simulink model "FCIACG_SIM"  (R2022a)
settings: Solver=VariableStepAuto  StartTime=0.0  StopTime=10.0  RelTol=1e-3
settings Model: Creator=Column  LastModifiedBy=Column

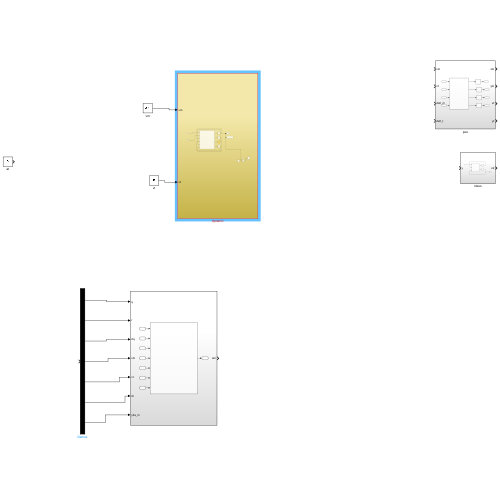
[thumbnail: Simulink's stored preview of the top-level diagram]
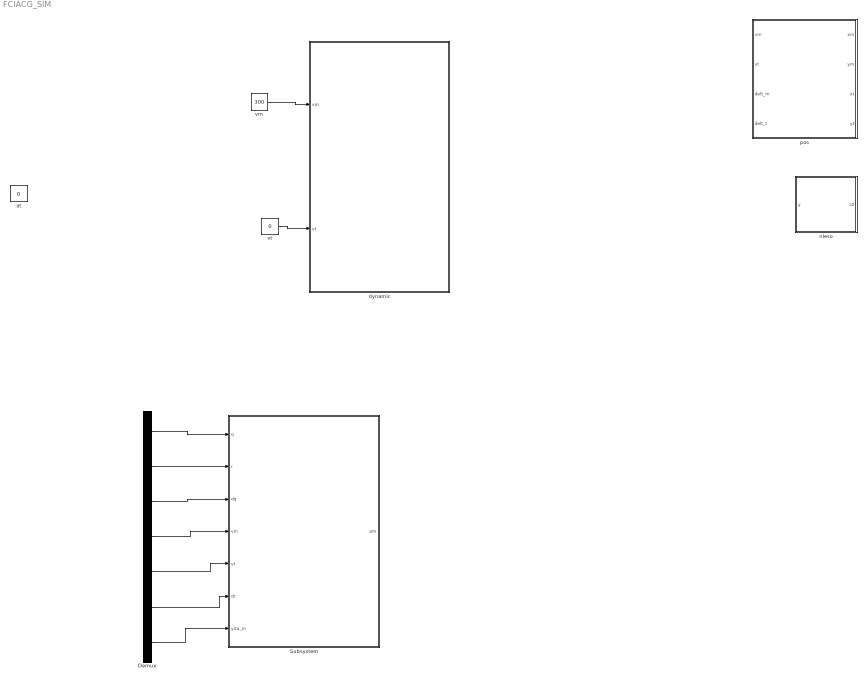
== system FCIACG_SIM ==
  Demux : Demux  Outputs=7
  Subsystem : Subsystem
  at : Constant  Value=0
  dynamic : Subsystem
  nleso : Subsystem
  pos : Subsystem
  vm : Constant  Value=300
  vt : Constant  Value=0
  wires:
  vm/1 -> dynamic/1(vm)
  Demux/1 -> Subsystem/1(q)
  Demux/2 -> Subsystem/2(r)
  Demux/3 -> Subsystem/3(dq)
  Demux/4 -> Subsystem/4(vm)
  Demux/5 -> Subsystem/5(vt)
  Demux/6 -> Subsystem/6(dr)
  Demux/7 -> Subsystem/7(yita_m)
  vt/1 -> dynamic/2(vt)

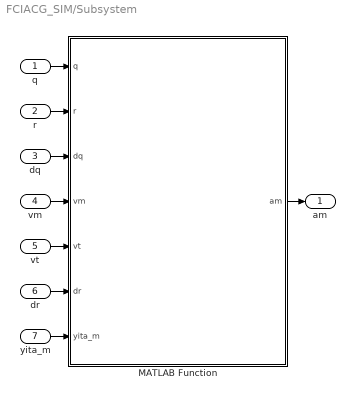
== system FCIACG_SIM/Subsystem ==
  q : Inport
  r : Inport  Port=2
  dq : Inport  Port=3
  vm : Inport  Port=4
  vt : Inport  Port=5
  dr : Inport  Port=6
  yita_m : Inport  Port=7
  MATLAB Function : MATLAB Function  TreatAsAtomicUnit=on
  am : Outport
  wires:
  MATLAB Function/1(am) -> am/1
  r/1 -> MATLAB Function/2(r)
  q/1 -> MATLAB Function/1(q)
  yita_m/1 -> MATLAB Function/7(yita_m)
  vt/1 -> MATLAB Function/5(vt)
  dr/1 -> MATLAB Function/6(dr)
  vm/1 -> MATLAB Function/4(vm)
  dq/1 -> MATLAB Function/3(dq)

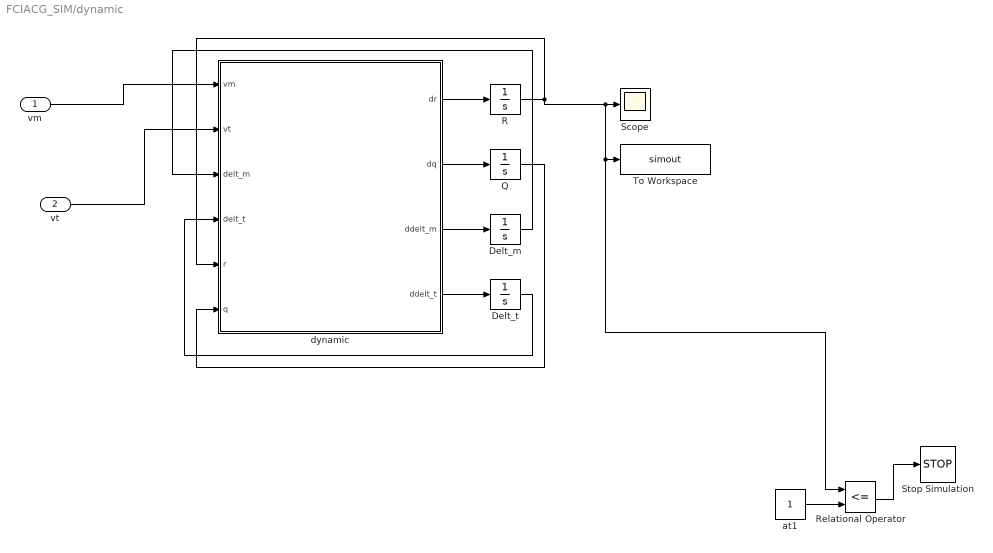
== system FCIACG_SIM/dynamic ==
  vm : Inport
  vt : Inport  Port=2
  Delt_m : Integrator
  Delt_t : Integrator
  Q : Integrator
  R : Integrator  InitialCondition=10000
  Relational Operator : RelationalOperator  Operator=<=  OutDataTypeStr=boolean  RndMeth=Simplest  InputSameDT=off
  Scope : Scope
  Stop Simulation : Stop
  To Workspace : ToWorkspace  VariableName=simout  SaveFormat=Timeseries  SampleTime=-1
  at1 : Constant
  dynamic : MATLAB Function  TreatAsAtomicUnit=on
  wires:
  dynamic/2(dq) -> Q/1
  vt/1 -> dynamic/2(vt)
  dynamic/3(ddelt_m) -> Delt_m/1
  dynamic/4(ddelt_t) -> Delt_t/1
  dynamic/1(dr) -> R/1
  vm/1 -> dynamic/1(vm)
  Q/1 -> dynamic/6(q)
  Delt_m/1 -> dynamic/3(delt_m)
  Delt_t/1 -> dynamic/4(delt_t)
  Relational Operator/1 -> Stop Simulation/1
  at1/1 -> Relational Operator/2
  R/1 -> Relational Operator/1, To Workspace/1, Scope/1, dynamic/5(r)

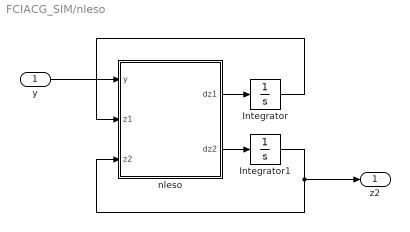
== system FCIACG_SIM/nleso ==
  y : Inport
  Integrator : Integrator
  Integrator1 : Integrator
  nleso : MATLAB Function  TreatAsAtomicUnit=on
  z2 : Outport
  wires:
  Integrator1/1 -> z2/1, nleso/3(z2)
  Integrator/1 -> nleso/2(z1)
  nleso/1(dz1) -> Integrator/1
  nleso/2(dz2) -> Integrator1/1
  y/1 -> nleso/1(y)

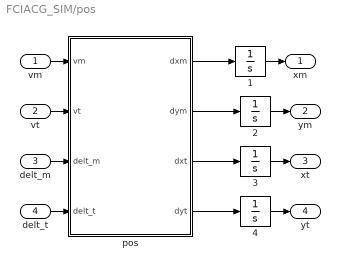
== system FCIACG_SIM/pos ==
  vm : Inport
  vt : Inport  Port=2
  delt_m : Inport  Port=3
  delt_t : Inport  Port=4
  {1..4} (4 alike) : Integrator
  pos : MATLAB Function  TreatAsAtomicUnit=on
  xm : Outport
  ym : Outport  Port=2
  xt : Outport  Port=3
  yt : Outport  Port=4
  wires:
  delt_t/1 -> pos/4(delt_t)
  1/1 -> xm/1
  delt_m/1 -> pos/3(delt_m)
  pos/1(dxm) -> 1/1
  3/1 -> xt/1
  pos/2(dym) -> 2/1
  vm/1 -> pos/1(vm)
  vt/1 -> pos/2(vt)
  2/1 -> ym/1
  pos/4(dyt) -> 4/1
  pos/3(dxt) -> 3/1
  4/1 -> yt/1

== matlab function FCIACG_SIM/pos/pos ==
  data: vm input; dxm output; vt input; delt_m input; delt_t input; dym output; dxt output; dyt output
function [dxm,dym,dxt,dyt] = fcn(vm,vt,delt_m,delt_t)


dxm = vm * cos(delt_m);

dym = vm * sin(delt_m);

dxt = vt * cos(delt_t);

dyt = vt * sin(delt_t);

end

== matlab function FCIACG_SIM/dynamic/dynamic ==
  data: vm input; dr output; vt input; delt_m input; delt_t input; dq output; ddelt_m output; ddelt_t output; r input; q input
function [dr,dq,ddelt_m,ddelt_t] = fcn(vm,vt,delt_m,delt_t,r,q)

yita_m = q - delt_m;

yita_t = q - delt_t;



dr = -vm * cos(yita_m) + vt * cos(yita_t);

dq = (vm * sin(yita_m) - vt *sin(yita_t)) /r;






yita_m_max = 45 * pi / 180; % 45
sigema = 0.1;
qd = -90 * pi / 180;
k1 = 2;

% 假如观测器之后这里需要进行改到k2
k2 = 0.2;

kc = vm * sin(yita_m_max) - vt;

x1 = q - qd;

x2 = r * dq;






m1 = ( -kc * abs(x1) / (abs(x1) + sigema)^2 + kc / (abs(x1) + sigema) -dr)*(x2/r);



da1 = ((-kc * abs(x1) / (abs(x1) + sigema)^2) - (kc / (abs(x1) + sigema))) * (x2/r);


w = (kc) / (abs(x1) + sigema);

a1 = -w *x1;
s = w * x1 + x2;

tmp_p = log((kc + s + a1) * (kc - a1) / ((kc -s -a1) * (kc +a1)));

p = kc * tmp_p /(2*s);


tmp_am = (-m1 - da1 + ((kc^2 - x2^2)/kc^2 * p * da1) - k1 *s - k2 * sign(s));


am = -1/(cos(yita_m)) * tmp_am;



ddelt_m = am / vm;

%ddelt_t = at / vt;

ddelt_t = 0;

== matlab function FCIACG_SIM/nleso/nleso ==
  data: y input; dz1 output; z1 input; z2 input; dz2 output
function [dz1,dz2] = fcn(y,z1,z2)

% yita gama (0,1) 
% a1 a2 >0
a1 = 2;
a2 = 1;
yita = 0.05;
gama = 0.75;
dz1 = z2 + a1 * (abs((y-z1)/yita))^gama * sign(y - z1);

dz2 = a2/yita * (abs((y-z1)/yita))^(2 * gama -1) * sign(y - z1);

end

== matlab function FCIACG_SIM/Subsystem/MATLAB Function ==
  data: q input; am output; r input; dq input; vm input; vt input; dr input; yita_m input
function am = fcn(q,r,dq,vm,vt,dr,yita_m)

% q r dq vm vt dr yita_m


yita_m_max = 45 * pi / 180; % 45
sigema = 0.1;
qd = -90 * pi / 180;
k1 = 2;

% 假如观测器之后这里需要进行改到k2
k2 = 0.2;

kc = vm * sin(yita_m_max) - vt;

x1 = q - qd;

x2 = r * dq;



m1 = ( -kc * abs(x1) / (abs(x1) + sigema)^2 + kc / (abs(x1) + sigema) -dr)*(x2/r);



da1 = ((-kc * abs(x1) / (abs(x1) + sigema)^2) - (kc / (abs(x1) + sigema))) * (x2/r);


w = (kc) / (abs(x1) + sigema);

a1 = -w *x1;
s = w * x1 + x2;

tmp_p = log((kc + s + a1) * (kc - a1) / ((kc -s -a1) * (kc +a1)));

p = kc * tmp_p /(2*s);


tmp_am = (-m1 - da1 + ((kc^2 - x2^2)/kc^2 * p * da1) - k1 *s - k2 * sign(s));


am = -1/(cos(yita_m)) * tmp_am;


end
